simulink model "swing_up"  (R2019b)
settings: Solver=VariableStepAuto  StartTime=0.0  StopTime=100  RelTol=1e-3
values from neighbouring files (symbols this model uses):
  c = 0.5    [params.m]
  dtheta1 = 400 * (2*pi/60)    (= 41.8879020479)    [params.m]
  Eo = 2*m*lcg*g    (= 0.836369208)    [params.m]
  g = 9.81    [params.m]
  Id = 0.0148    [params.m]
  J1 = 0.1314    [params.m]
  Jz_bar = 0.0131    [params.m]
  lcg = 0.2698    [params.m]
  m = 0.1580    (= 0.158)    [params.m]
  rh = 0.37    [params.m]
undefined symbols (not defined in the file or in its folder): dth1, k
settings Model: Creator=Nilpa  LastModifiedBy=Nilpa

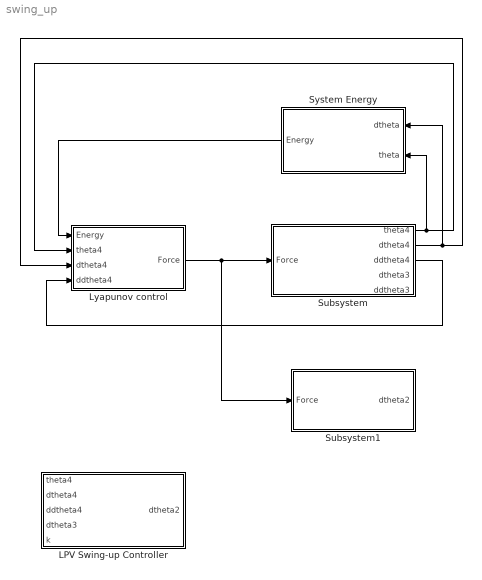
== system swing_up ==
  LPV Swing-up Controller : Subsystem
  Lyapunov control : Subsystem
  Subsystem : Subsystem
  Subsystem1 : Subsystem
  System Energy : Subsystem
  wires:
  Subsystem/1(theta4) -> Lyapunov control/2(theta4), System Energy/2(theta)
  Subsystem/2(dtheta4) -> Lyapunov control/3(dtheta4), System Energy/1(dtheta)
  Lyapunov control/1(Force) -> Subsystem1/1(Force), Subsystem/1(Force)
  System Energy/1(Energy) -> Lyapunov control/1(Energy)
  Subsystem/3(ddtheta4) -> Lyapunov control/4(ddtheta4)

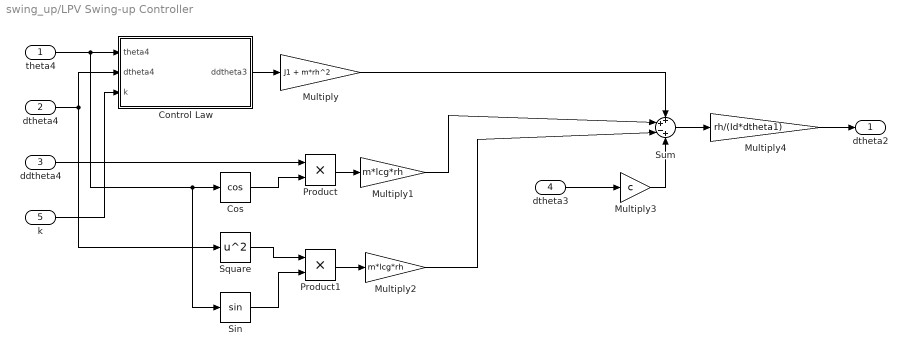
== system swing_up/LPV Swing-up Controller ==
  theta4 : Inport
  dtheta4 : Inport  Port=2
  ddtheta4 : Inport  Port=3
  dtheta3 : Inport  Port=4
  k : Inport  Port=5
  Control Law : Subsystem
  Cos : Trigonometry  Operator=cos
  Multiply : Gain  Gain=J1 + m*rh^2
  Multiply1 : Gain  Gain=m*lcg*rh
  Multiply2 : Gain  Gain=m*lcg*rh
  Multiply3 : Gain  Gain=c
  Multiply4 : Gain  Gain=rh/(Id*dtheta1)
  Product : Product
  Product1 : Product
  Sin : Trigonometry
  Square : Math  Operator=square  SignedPower=off  SaturateOnIntegerOverflow=on
  Sum : Sum  Inputs=++-+
  dtheta2 : Outport
  wires:
  theta4/1 -> Control Law/1(theta4), Sin/1, Cos/1
  dtheta4/1 -> Square/1, Control Law/2(dtheta4)
  k/1 -> Control Law/3(k)
  Control Law/1(ddtheta3) -> Multiply/1
  Multiply/1 -> Sum/1
  Cos/1 -> Product/2
  ddtheta4/1 -> Product/1
  Product/1 -> Multiply1/1
  Multiply1/1 -> Sum/2
  Sin/1 -> Product1/2
  Square/1 -> Product1/1
  Product1/1 -> Multiply2/1
  Multiply2/1 -> Sum/3
  Multiply3/1 -> Sum/4
  Sum/1 -> Multiply4/1
  Multiply4/1 -> dtheta2/1
  dtheta3/1 -> Multiply3/1

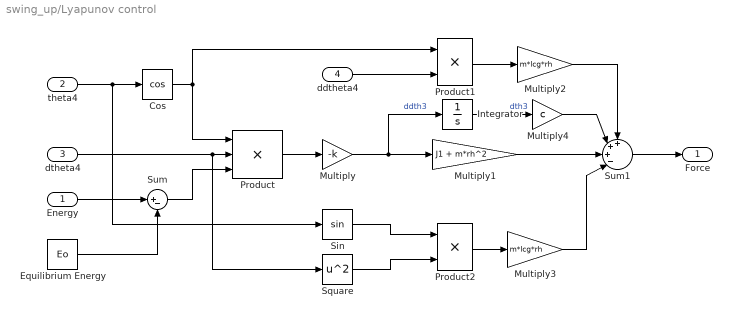
== system swing_up/Lyapunov control ==
  Energy : Inport
  theta4 : Inport  Port=2
  dtheta4 : Inport  Port=3
  ddtheta4 : Inport  Port=4
  Cos : Trigonometry  Operator=cos
  Equilibrium Energy : Constant  Value=Eo
  Integrator : Integrator
  Multiply : Gain  Gain=-k
  Multiply1 : Gain  Gain=J1 + m*rh^2
  Multiply2 : Gain  Gain=m*lcg*rh
  Multiply3 : Gain  Gain=m*lcg*rh
  Multiply4 : Gain  Gain=c
  Product : Product  Inputs=3
  Product1 : Product
  Product2 : Product
  Sin : Trigonometry
  Square : Math  Operator=square  SignedPower=off  SaturateOnIntegerOverflow=on
  Sum : Sum  Inputs=|+-
  Sum1 : Sum  Inputs=+++-|
  Force : Outport
  wires:
  Product/1 -> Multiply/1
  theta4/1 -> Cos/1, Sin/1
  Cos/1 -> Product/1, Product1/1
  dtheta4/1 -> Square/1, Product/2
  Energy/1 -> Sum/1
  Sum/1 -> Product/3
  Equilibrium Energy/1 -> Sum/2
  Multiply/1 -> Integrator/1, Multiply1/1  "ddth3"
  Multiply1/1 -> Sum1/3
  Sum1/1 -> Force/1
  Product1/1 -> Multiply2/1
  Multiply2/1 -> Sum1/1
  Sin/1 -> Product2/1
  Square/1 -> Product2/2
  Product2/1 -> Multiply3/1
  Multiply3/1 -> Sum1/4
  ddtheta4/1 -> Product1/2
  Integrator/1 -> Multiply4/1  "dth3"
  Multiply4/1 -> Sum1/2

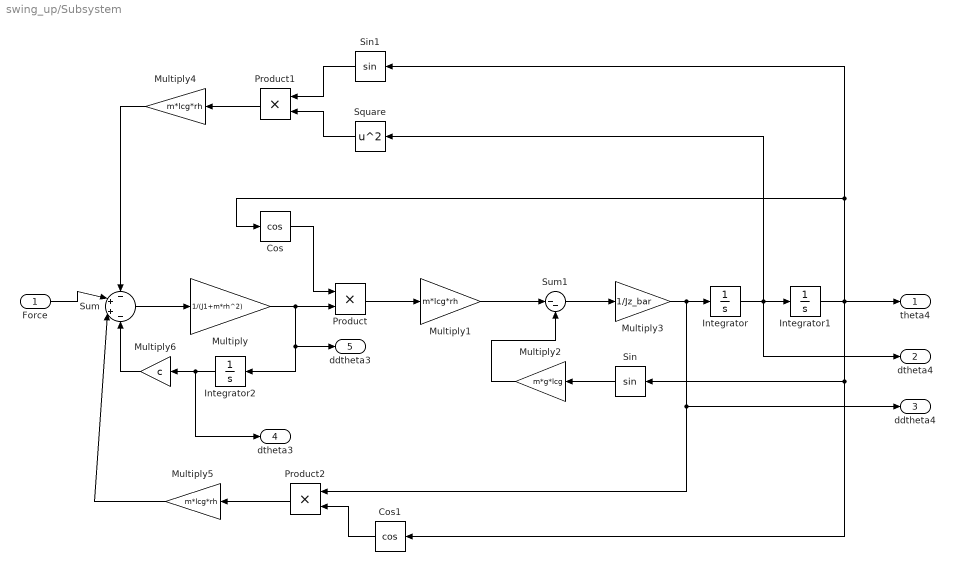
== system swing_up/Subsystem ==
  Force : Inport
  Cos : Trigonometry  Operator=cos
  Cos1 : Trigonometry  Operator=cos
  Integrator : Integrator
  Integrator1 : Integrator
  Integrator2 : Integrator
  Multiply : Gain  Gain=1/(J1+m*rh^2)
  Multiply1 : Gain  Gain=m*lcg*rh
  Multiply2 : Gain  Gain=m*g*lcg
  Multiply3 : Gain  Gain=1/Jz_bar
  Multiply4 : Gain  Gain=m*lcg*rh
  Multiply5 : Gain  Gain=m*lcg*rh
  Multiply6 : Gain  Gain=c
  Product : Product
  Product1 : Product
  Product2 : Product
  Sin : Trigonometry
  Sin1 : Trigonometry
  Square : Math  Operator=square  SignedPower=off  SaturateOnIntegerOverflow=on
  Sum : Sum  Inputs=-++-
  Sum1 : Sum  Inputs=|--
  theta4 : Outport
  dtheta4 : Outport  Port=2
  ddtheta4 : Outport  Port=3
  dtheta3 : Outport  Port=4
  ddtheta3 : Outport  Port=5
  wires:
  Force/1 -> Sum/2
  Sum/1 -> Multiply/1
  Multiply/1 -> Integrator2/1, ddtheta3/1, Product/2
  Cos/1 -> Product/1
  Product/1 -> Multiply1/1
  Multiply1/1 -> Sum1/1
  Sin/1 -> Multiply2/1
  Multiply2/1 -> Sum1/2
  Sum1/1 -> Multiply3/1
  Multiply3/1 -> ddtheta4/1, Product2/1, Integrator/1
  Integrator/1 -> dtheta4/1, Square/1, Integrator1/1
  Integrator1/1 -> Cos1/1, Sin/1, theta4/1, Cos/1, Sin1/1
  Product1/1 -> Multiply4/1
  Multiply4/1 -> Sum/1
  Sin1/1 -> Product1/1
  Square/1 -> Product1/2
  Product2/1 -> Multiply5/1
  Multiply5/1 -> Sum/3
  Cos1/1 -> Product2/2
  Integrator2/1 -> Multiply6/1, dtheta3/1
  Multiply6/1 -> Sum/4

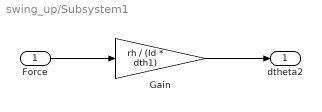
== system swing_up/Subsystem1 ==
  Force : Inport
  Gain : Gain  Gain=rh / (Id * dth1)
  dtheta2 : Outport
  wires:
  Force/1 -> Gain/1
  Gain/1 -> dtheta2/1

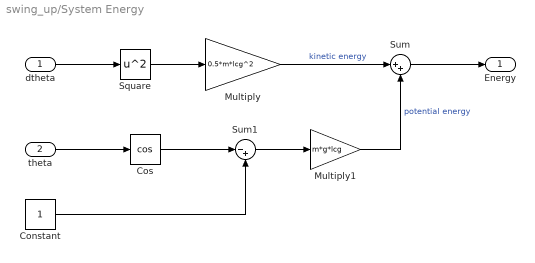
== system swing_up/System Energy ==
  dtheta : Inport
  theta : Inport  Port=2
  Constant : Constant
  Cos : Trigonometry  Operator=cos
  Multiply : Gain  Gain=0.5*m*lcg^2
  Multiply1 : Gain  Gain=m*g*lcg
  Square : Math  Operator=square  SignedPower=off  SaturateOnIntegerOverflow=on
  Sum : Sum  Inputs=|++
  Sum1 : Sum  Inputs=|-+
  Energy : Outport
  wires:
  Sum/1 -> Energy/1
  Multiply/1 -> Sum/1  "kinetic energy"
  Square/1 -> Multiply/1
  dtheta/1 -> Square/1
  Constant/1 -> Sum1/2
  Cos/1 -> Sum1/1
  theta/1 -> Cos/1
  Sum1/1 -> Multiply1/1
  Multiply1/1 -> Sum/2  "potential energy"

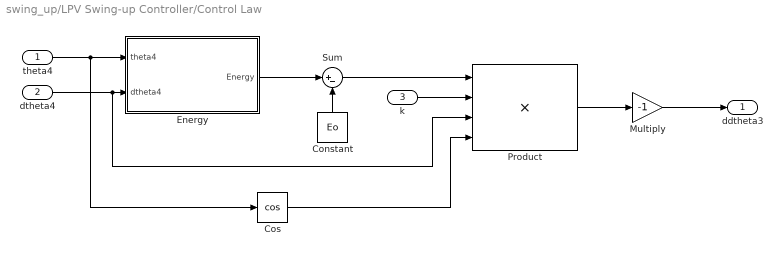
== system swing_up/LPV Swing-up Controller/Control Law ==
  theta4 : Inport
  dtheta4 : Inport  Port=2
  k : Inport  Port=3
  Constant : Constant  Value=Eo
  Cos : Trigonometry  Operator=cos
  Energy : Subsystem
  Multiply : Gain  Gain=-1
  Product : Product  Inputs=4
  Sum : Sum  Inputs=|+-
  ddtheta3 : Outport
  wires:
  Energy/1(Energy) -> Sum/1
  Constant/1 -> Sum/2
  theta4/1 -> Cos/1, Energy/1(theta4)
  dtheta4/1 -> Product/3, Energy/2(dtheta4)
  Sum/1 -> Product/1
  k/1 -> Product/2
  Multiply/1 -> ddtheta3/1
  Product/1 -> Multiply/1
  Cos/1 -> Product/4

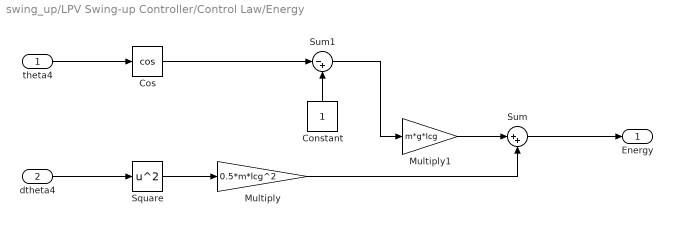
== system swing_up/LPV Swing-up Controller/Control Law/Energy ==
  theta4 : Inport
  dtheta4 : Inport  Port=2
  Constant : Constant
  Cos : Trigonometry  Operator=cos
  Multiply : Gain  Gain=0.5*m*lcg^2
  Multiply1 : Gain  Gain=m*g*lcg
  Square : Math  Operator=square  SignedPower=off  SaturateOnIntegerOverflow=on
  Sum : Sum  Inputs=|++
  Sum1 : Sum  Inputs=|-+
  Energy : Outport
  wires:
  dtheta4/1 -> Square/1
  Square/1 -> Multiply/1
  Multiply/1 -> Sum/2
  Sum/1 -> Energy/1
  theta4/1 -> Cos/1
  Cos/1 -> Sum1/1
  Constant/1 -> Sum1/2
  Multiply1/1 -> Sum/1
  Sum1/1 -> Multiply1/1
